simulink model "mylib"  (R2016b)
settings: Solver=FixedStepAuto  StartTime=0.0  StopTime=10.0  RelTol=1e-3  SampleTimeConstraint=STIndependent
settings Model: Creator=Colin  LastModifiedBy=Colin

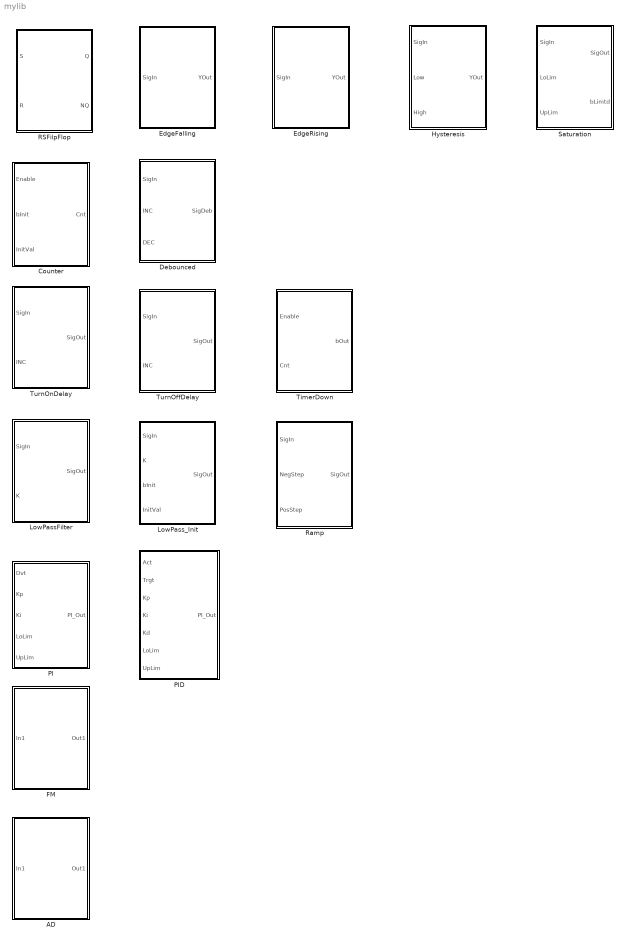
== system mylib ==
  AD : Subsystem
  Counter : Subsystem
  Debounced : Subsystem
  EdgeFalling : Subsystem
  EdgeRising : Subsystem
  FM : Subsystem
  Hysteresis : Subsystem
  LowPassFilter : Subsystem
  LowPass_Init : Subsystem
  PI : Subsystem
  PID : Subsystem
  RSFilpFlop : Subsystem
  Ramp : Subsystem
  Saturation : Subsystem
  TimerDown : Subsystem
  TurnOffDelay : Subsystem
  TurnOnDelay : Subsystem

== system mylib/AD ==
  In1 : Inport
  Out1 : Outport

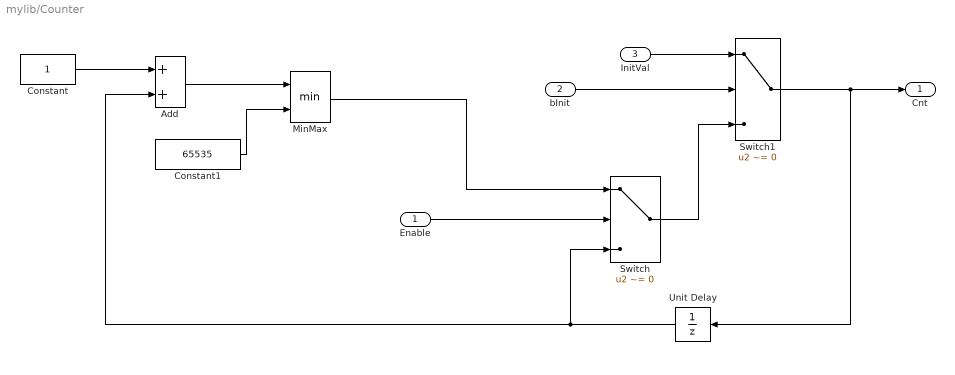
== system mylib/Counter ==
  Enable : Inport
  bInit : Inport  Port=2
  InitVal : Inport  Port=3
  Add : Sum
  Constant : Constant
  Constant1 : Constant  Value=65535
  MinMax : MinMax  Inputs=2
  Switch : Switch  Criteria=u2 ~= 0
  Switch1 : Switch  Criteria=u2 ~= 0
  Unit Delay : UnitDelay  SampleTime=-1
      settings: AttributesFormatString=InitialValue=%<InitialCondition>
  Cnt : Outport
  wires:
  Enable/1 -> Switch/2
  Add/1 -> MinMax/1
  MinMax/1 -> Switch/1
  Constant1/1 -> MinMax/2
  Switch1/1 -> Unit Delay/1, Cnt/1
  bInit/1 -> Switch1/2
  InitVal/1 -> Switch1/1
  Switch/1 -> Switch1/3
  Constant/1 -> Add/1
  Unit Delay/1 -> Switch/3, Add/2

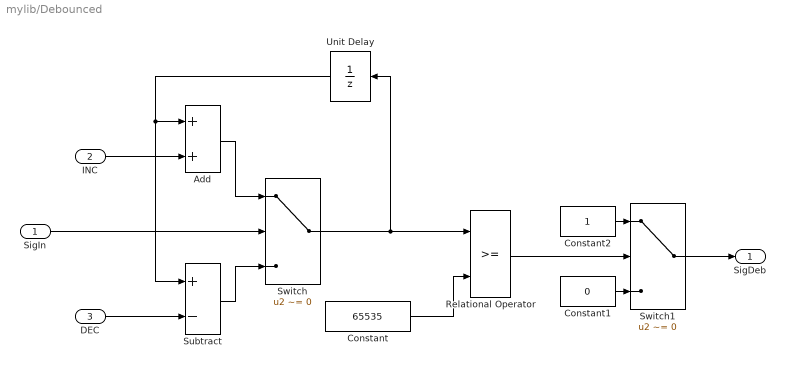
== system mylib/Debounced ==
  SigIn : Inport  OutDataTypeStr=boolean
  INC : Inport  Port=2
  DEC : Inport  Port=3
  Add : Sum
  Constant : Constant  Value=65535
  Constant1 : Constant  Value=0  OutDataTypeStr=boolean
  Constant2 : Constant  OutDataTypeStr=boolean
  Relational Operator : RelationalOperator  OutDataTypeStr=boolean  RndMeth=Simplest
  Subtract : Sum  Inputs=+-
  Switch : Switch  Criteria=u2 ~= 0
  Switch1 : Switch  Criteria=u2 ~= 0
  Unit Delay : UnitDelay  SampleTime=-1
      settings: AttributesFormatString=InitialValue=%<InitialCondition>
  SigDeb : Outport  OutDataTypeStr=boolean
  wires:
  SigIn/1 -> Switch/2
  Switch/1 -> Unit Delay/1, Relational Operator/1
  Constant/1 -> Relational Operator/2
  Relational Operator/1 -> Switch1/2
  Switch1/1 -> SigDeb/1
  Constant1/1 -> Switch1/3
  Constant2/1 -> Switch1/1
  INC/1 -> Add/2
  Unit Delay/1 -> Subtract/1, Add/1
  Add/1 -> Switch/1
  Subtract/1 -> Switch/3
  DEC/1 -> Subtract/2

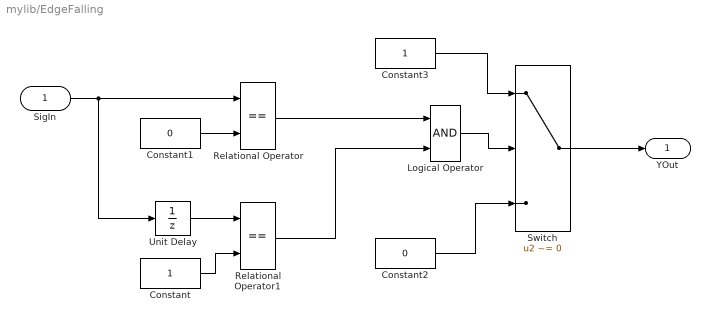
== system mylib/EdgeFalling ==
  SigIn : Inport  OutDataTypeStr=boolean
  Constant : Constant  OutDataTypeStr=boolean
  Constant1 : Constant  Value=0  OutDataTypeStr=boolean
  Constant2 : Constant  Value=0  OutDataTypeStr=boolean
  Constant3 : Constant  OutDataTypeStr=boolean
  Logical Operator : Logic  AllPortsSameDT=off  OutDataTypeStr=boolean
  Relational Operator : RelationalOperator  Operator===  OutDataTypeStr=boolean  RndMeth=Simplest
  Relational Operator1 : RelationalOperator  Operator===  OutDataTypeStr=boolean  RndMeth=Simplest
  Switch : Switch  Criteria=u2 ~= 0
  Unit Delay : UnitDelay  SampleTime=-1
      settings: AttributesFormatString=InitialValue=%<InitialCondition>
  YOut : Outport  OutDataTypeStr=boolean
  wires:
  Logical Operator/1 -> Switch/2
  Switch/1 -> YOut/1
  SigIn/1 -> Unit Delay/1, Relational Operator/1
  Constant1/1 -> Relational Operator/2
  Constant/1 -> Relational Operator1/2
  Unit Delay/1 -> Relational Operator1/1
  Relational Operator/1 -> Logical Operator/1
  Relational Operator1/1 -> Logical Operator/2
  Constant2/1 -> Switch/3
  Constant3/1 -> Switch/1

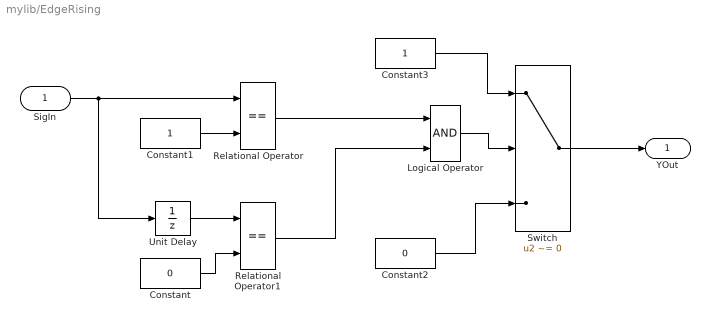
== system mylib/EdgeRising ==
  SigIn : Inport  OutDataTypeStr=boolean
  Constant : Constant  Value=0  OutDataTypeStr=boolean
  Constant1 : Constant  OutDataTypeStr=boolean
  Constant2 : Constant  Value=0  OutDataTypeStr=boolean
  Constant3 : Constant  OutDataTypeStr=boolean
  Logical Operator : Logic  AllPortsSameDT=off  OutDataTypeStr=boolean
  Relational Operator : RelationalOperator  Operator===  OutDataTypeStr=boolean  RndMeth=Simplest
  Relational Operator1 : RelationalOperator  Operator===  OutDataTypeStr=boolean  RndMeth=Simplest
  Switch : Switch  Criteria=u2 ~= 0
  Unit Delay : UnitDelay  SampleTime=-1
      settings: AttributesFormatString=InitialValue=%<InitialCondition>
  YOut : Outport  OutDataTypeStr=boolean
  wires:
  Logical Operator/1 -> Switch/2
  Switch/1 -> YOut/1
  SigIn/1 -> Unit Delay/1, Relational Operator/1
  Constant1/1 -> Relational Operator/2
  Constant/1 -> Relational Operator1/2
  Unit Delay/1 -> Relational Operator1/1
  Relational Operator/1 -> Logical Operator/1
  Relational Operator1/1 -> Logical Operator/2
  Constant2/1 -> Switch/3
  Constant3/1 -> Switch/1

== system mylib/FM ==
  In1 : Inport
  Out1 : Outport

== system mylib/Hysteresis ==
  SigIn : Inport
  Low : Inport  Port=2
  High : Inport  Port=3
  Constant : Constant  OutDataTypeStr=boolean
  Constant1 : Constant  Value=0  OutDataTypeStr=boolean
  Delay : Delay  DelayLength=1  InitialCondition=0
      settings: AttributesFormatString=InitialValue=%<InitialCondition>
  Relational Operator : RelationalOperator  Operator=>  OutDataTypeStr=boolean  RndMeth=Nearest  InputSameDT=on
  Relational Operator1 : RelationalOperator  Operator=<  OutDataTypeStr=boolean  RndMeth=Nearest  InputSameDT=on
  Switch : Switch  Criteria=u2 ~= 0  InputSameDT=on
  Switch1 : Switch  Criteria=u2 ~= 0  InputSameDT=on
  YOut : Outport  OutDataTypeStr=boolean
  wires:
  SigIn/1 -> Relational Operator/1, Relational Operator1/1
  High/1 -> Relational Operator/2
  Relational Operator/1 -> Switch/2
  Constant/1 -> Switch/1
  Switch1/1 -> Switch/3
  Relational Operator1/1 -> Switch1/2
  Low/1 -> Relational Operator1/2
  Constant1/1 -> Switch1/1
  Switch/1 -> YOut/1, Delay/1
  Delay/1 -> Switch1/3

== system mylib/LowPassFilter ==
  SigIn : Inport  SampleTime=0.01
  K : Inport  Port=2  SampleTime=0.01
  Product : Product
  Subtract1 : Sum  Inputs=+-
  Sum : Sum  Inputs=+|+
  Unit Delay : UnitDelay  SampleTime=-1
      settings: AttributesFormatString=InitialValue=%<InitialCondition>
  SigOut : Outport  SampleTime=0.01
  wires:
  K/1 -> Product/1
  SigIn/1 -> Subtract1/1
  Unit Delay/1 -> Sum/2, Subtract1/2
  Subtract1/1 -> Product/2
  Product/1 -> Sum/1
  Sum/1 -> Unit Delay/1, SigOut/1

== system mylib/LowPass_Init ==
  SigIn : Inport  SampleTime=0.01
  K : Inport  Port=2  SampleTime=0.01
  bInit : Inport  Port=3  SampleTime=0.01
  InitVal : Inport  Port=4  SampleTime=0.01
  Product : Product
  Subtract1 : Sum  Inputs=+-
  Sum : Sum  Inputs=+|+
  Switch : Switch  Criteria=u2 ~= 0
  Unit Delay : UnitDelay  SampleTime=-1
      settings: AttributesFormatString=InitialValue=%<InitialCondition>
  SigOut : Outport  SampleTime=0.01
  wires:
  K/1 -> Product/1
  SigIn/1 -> Subtract1/1
  Unit Delay/1 -> Sum/2, Subtract1/2
  Subtract1/1 -> Product/2
  Product/1 -> Sum/1
  Sum/1 -> Switch/3
  Switch/1 -> Unit Delay/1, SigOut/1
  bInit/1 -> Switch/2
  InitVal/1 -> Switch/1

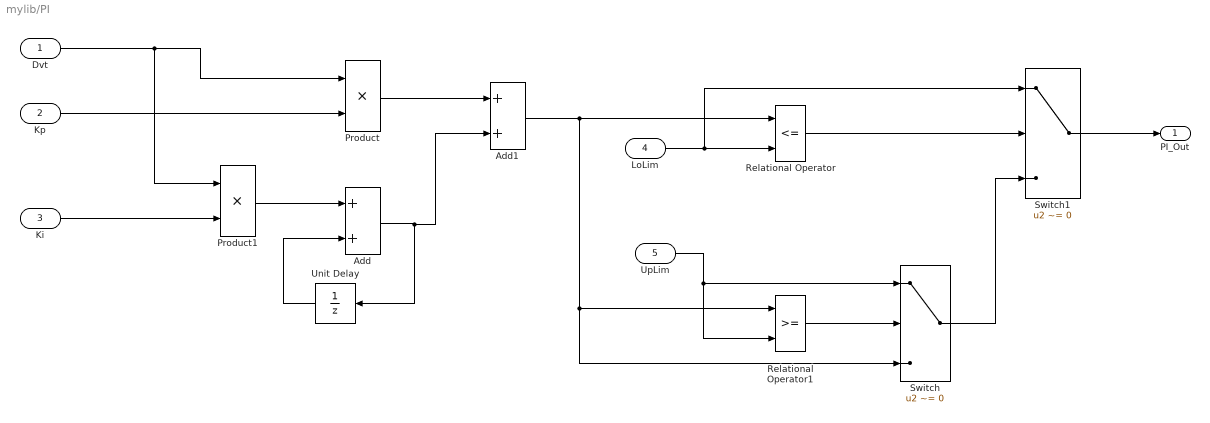
== system mylib/PI ==
  Dvt : Inport
  Kp : Inport  Port=2
  Ki : Inport  Port=3
  LoLim : Inport  Port=4
  UpLim : Inport  Port=5
  Add : Sum
  Add1 : Sum
  Product : Product
  Product1 : Product
  Relational Operator : RelationalOperator  Operator=<=  OutDataTypeStr=boolean  RndMeth=Simplest  InputSameDT=on
  Relational Operator1 : RelationalOperator  OutDataTypeStr=boolean  RndMeth=Simplest  InputSameDT=on
  Switch : Switch  Criteria=u2 ~= 0
  Switch1 : Switch  Criteria=u2 ~= 0
  Unit Delay : UnitDelay  SampleTime=-1
      settings: AttributesFormatString=InitialValue=%<InitialCondition>
  PI_Out : Outport
  wires:
  Dvt/1 -> Product/1, Product1/1
  Kp/1 -> Product/2
  Ki/1 -> Product1/2
  Product1/1 -> Add/1
  Add/1 -> Add1/2, Unit Delay/1
  Unit Delay/1 -> Add/2
  Product/1 -> Add1/1
  Add1/1 -> Relational Operator/1, Switch/3, Relational Operator1/1
  UpLim/1 -> Relational Operator1/2, Switch/1
  LoLim/1 -> Switch1/1, Relational Operator/2
  Relational Operator/1 -> Switch1/2
  Relational Operator1/1 -> Switch/2
  Switch/1 -> Switch1/3
  Switch1/1 -> PI_Out/1

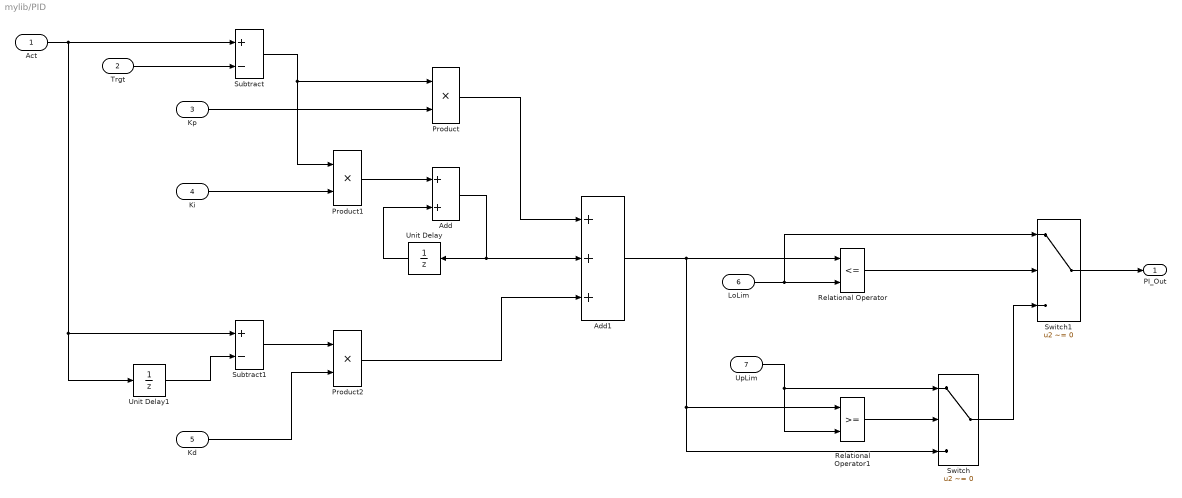
== system mylib/PID ==
  Act : Inport
  Trgt : Inport  Port=2
  Kp : Inport  Port=3
  Ki : Inport  Port=4
  Kd : Inport  Port=5
  LoLim : Inport  Port=6
  UpLim : Inport  Port=7
  Add : Sum
  Add1 : Sum  Inputs=+++
  Product : Product
  Product1 : Product
  Product2 : Product
  Relational Operator : RelationalOperator  Operator=<=  OutDataTypeStr=boolean  RndMeth=Simplest  InputSameDT=on
  Relational Operator1 : RelationalOperator  OutDataTypeStr=boolean  RndMeth=Simplest  InputSameDT=on
  Subtract : Sum  Inputs=+-
  Subtract1 : Sum  Inputs=+-
  Switch : Switch  Criteria=u2 ~= 0
  Switch1 : Switch  Criteria=u2 ~= 0
  Unit Delay : UnitDelay  SampleTime=-1
      settings: AttributesFormatString=InitialValue=%<InitialCondition>
  Unit Delay1 : UnitDelay  SampleTime=-1
      settings: AttributesFormatString=InitialValue=%<InitialCondition>
  PI_Out : Outport
  wires:
  Kp/1 -> Product/2
  Ki/1 -> Product1/2
  Product1/1 -> Add/1
  Add/1 -> Unit Delay/1, Add1/2
  Unit Delay/1 -> Add/2
  Product/1 -> Add1/1
  Add1/1 -> Switch/3, Relational Operator1/1, Relational Operator/1
  UpLim/1 -> Relational Operator1/2, Switch/1
  LoLim/1 -> Switch1/1, Relational Operator/2
  Relational Operator/1 -> Switch1/2
  Relational Operator1/1 -> Switch/2
  Switch/1 -> Switch1/3
  Switch1/1 -> PI_Out/1
  Act/1 -> Unit Delay1/1, Subtract1/1, Subtract/1
  Trgt/1 -> Subtract/2
  Subtract/1 -> Product1/1, Product/1
  Unit Delay1/1 -> Subtract1/2
  Subtract1/1 -> Product2/1
  Kd/1 -> Product2/2
  Product2/1 -> Add1/3

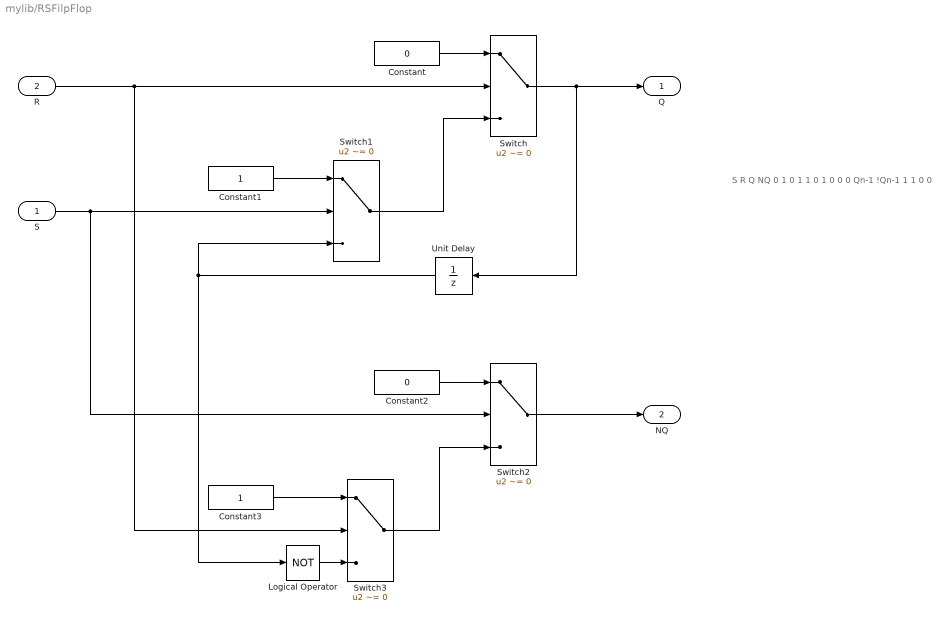
== system mylib/RSFilpFlop ==
  note: S
      | R
      | Q
      | NQ
      |
      | 0
      | 1
      | 0
      | 1
      |
      | 1
      | 0
      | 1
      | 0
      |
      | 0
      | 0
      | Qn-1
      | !Qn-1
      |
      | 1
      | 1
      | 0
      | 0
  S : Inport
  R : Inport  Port=2
  Constant : Constant  Value=0
  Constant1 : Constant
  Constant2 : Constant  Value=0
  Constant3 : Constant
  Logical Operator : Logic  Operator=NOT  AllPortsSameDT=off  OutDataTypeStr=boolean
  Switch{,1..3} (4 alike) : Switch  Criteria=u2 ~= 0
  Unit Delay : UnitDelay  SampleTime=-1
  Q : Outport
  NQ : Outport  Port=2
  wires:
  R/1 -> Switch3/2, Switch/2
  Constant/1 -> Switch/1
  Switch/1 -> Unit Delay/1, Q/1
  S/1 -> Switch2/2, Switch1/2
  Constant1/1 -> Switch1/1
  Switch1/1 -> Switch/3
  Unit Delay/1 -> Switch1/3, Logical Operator/1
  Switch2/1 -> NQ/1
  Constant2/1 -> Switch2/1
  Switch3/1 -> Switch2/3
  Constant3/1 -> Switch3/1
  Logical Operator/1 -> Switch3/3

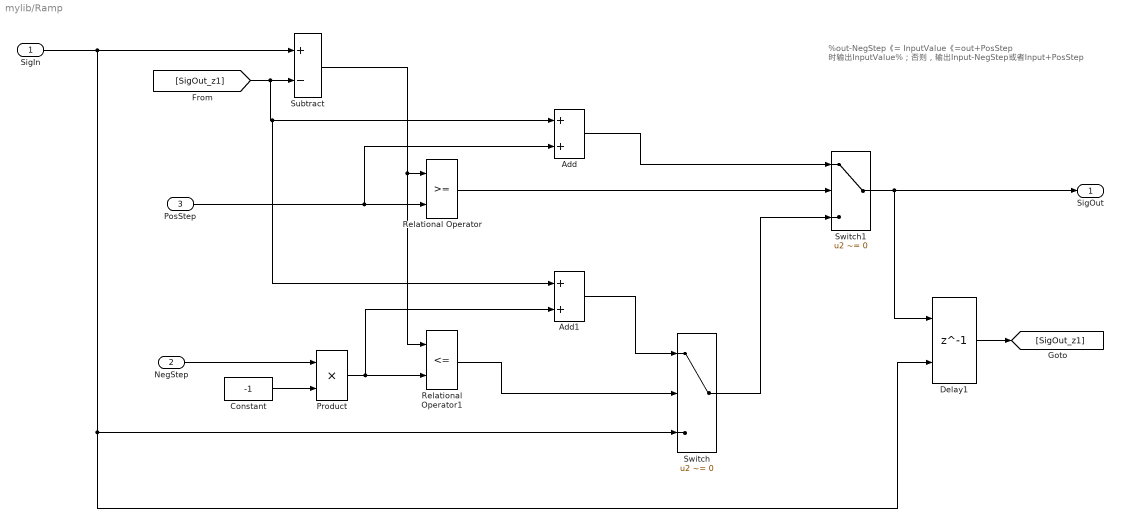
== system mylib/Ramp ==
  note: %out-NegStep《= InputValue《=out+PosStep
      | 时输出InputValue%；否则，输出Input-NegStep或者Input+PosStep
  SigIn : Inport
  NegStep : Inport  Port=2
  PosStep : Inport  Port=3
  Add : Sum
  Add1 : Sum
  Constant : Constant  Value=-1
  Delay1 : Delay  DelayLength=1  InitialConditionSource=Input port
      settings: InputPortMap=u0,p4
  Product : Product
  Relational Operator : RelationalOperator  OutDataTypeStr=boolean  RndMeth=Simplest
  Relational Operator1 : RelationalOperator  Operator=<=  OutDataTypeStr=boolean  RndMeth=Simplest
  Subtract : Sum  Inputs=+-
  Switch : Switch  Criteria=u2 ~= 0
  Switch1 : Switch  Criteria=u2 ~= 0
  SigOut : Outport
  wires:
  SigIn/1 -> Delay1/2, Switch/3, Subtract/1
  Subtract/1 -> Relational Operator1/1, Relational Operator/1
  PosStep/1 -> Add/2, Relational Operator/2
  Relational Operator/1 -> Switch1/2
  Switch1/1 -> Delay1/1, SigOut/1
  Add/1 -> Switch1/1
  Relational Operator1/1 -> Switch/2
  NegStep/1 -> Product/1
  Product/1 -> Add1/2, Relational Operator1/2
  Constant/1 -> Product/2
  Switch/1 -> Switch1/3
  Add1/1 -> Switch/1
  Delay1/1 -> [SigOut_z1]
  [SigOut_z1] -> Add1/1, Add/1, Subtract/2

== system mylib/Saturation ==
  SigIn : Inport
  LoLim : Inport  Port=2
  UpLim : Inport  Port=3
  Logical Operator : Logic  Operator=OR  AllPortsSameDT=off  OutDataTypeStr=boolean
  Relational Operator : RelationalOperator  Operator=<=  OutDataTypeStr=boolean  RndMeth=Simplest  InputSameDT=on
  Relational Operator1 : RelationalOperator  OutDataTypeStr=boolean  RndMeth=Simplest  InputSameDT=on
  Switch : Switch  Criteria=u2 ~= 0
  Switch1 : Switch  Criteria=u2 ~= 0
  SigOut : Outport
  bLimtd : Outport  Port=2  OutDataTypeStr=boolean
  wires:
  SigIn/1 -> Relational Operator/1, Switch/3, Relational Operator1/1
  UpLim/1 -> Relational Operator1/2, Switch/1
  LoLim/1 -> Switch1/1, Relational Operator/2
  Relational Operator/1 -> Logical Operator/1, Switch1/2
  Relational Operator1/1 -> Logical Operator/2, Switch/2
  Logical Operator/1 -> bLimtd/1
  Switch/1 -> Switch1/3
  Switch1/1 -> SigOut/1

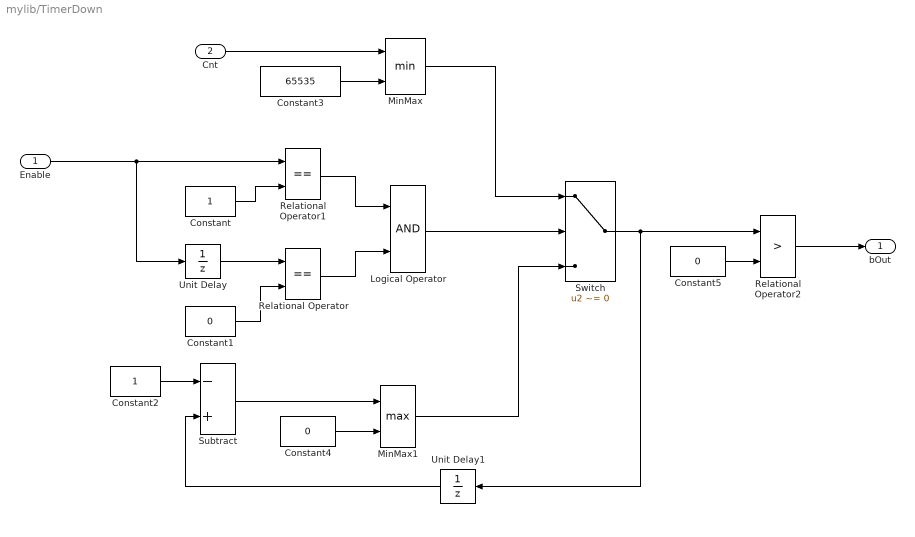
== system mylib/TimerDown ==
  Enable : Inport  OutDataTypeStr=boolean
  Cnt : Inport  Port=2
  Constant : Constant
  Constant1 : Constant  Value=0
  Constant2 : Constant
  Constant3 : Constant  Value=65535
  Constant4 : Constant  Value=0
  Constant5 : Constant  Value=0
  Logical Operator : Logic  AllPortsSameDT=off  OutDataTypeStr=boolean
  MinMax : MinMax  Inputs=2
  MinMax1 : MinMax  Function=max  Inputs=2
  Relational Operator : RelationalOperator  Operator===  OutDataTypeStr=boolean  RndMeth=Simplest
  Relational Operator1 : RelationalOperator  Operator===  OutDataTypeStr=boolean  RndMeth=Simplest
  Relational Operator2 : RelationalOperator  Operator=>  OutDataTypeStr=boolean  RndMeth=Simplest
  Subtract : Sum  Inputs=-+
  Switch : Switch  Criteria=u2 ~= 0
  Unit Delay : UnitDelay  SampleTime=-1
  Unit Delay1 : UnitDelay  SampleTime=-1
      settings: AttributesFormatString=InitialValue=%<InitialCondition>
  bOut : Outport  OutDataTypeStr=boolean
  wires:
  Enable/1 -> Unit Delay/1, Relational Operator1/1
  Unit Delay/1 -> Relational Operator/1
  Constant/1 -> Relational Operator1/2
  Constant1/1 -> Relational Operator/2
  Relational Operator1/1 -> Logical Operator/1
  Relational Operator/1 -> Logical Operator/2
  Logical Operator/1 -> Switch/2
  Cnt/1 -> MinMax/1
  Constant3/1 -> MinMax/2
  MinMax/1 -> Switch/1
  Constant2/1 -> Subtract/1
  Switch/1 -> Relational Operator2/1, Unit Delay1/1
  Unit Delay1/1 -> Subtract/2
  MinMax1/1 -> Switch/3
  Subtract/1 -> MinMax1/1
  Constant4/1 -> MinMax1/2
  Relational Operator2/1 -> bOut/1
  Constant5/1 -> Relational Operator2/2

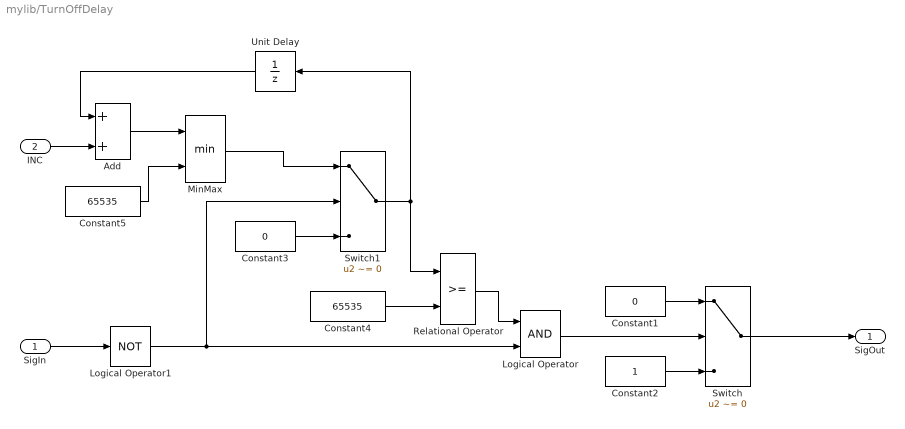
== system mylib/TurnOffDelay ==
  SigIn : Inport  OutDataTypeStr=boolean
  INC : Inport  Port=2
  Add : Sum
  Constant1 : Constant  Value=0
  Constant2 : Constant
  Constant3 : Constant  Value=0
  Constant4 : Constant  Value=65535
  Constant5 : Constant  Value=65535
  Logical Operator : Logic  AllPortsSameDT=off  OutDataTypeStr=boolean
  Logical Operator1 : Logic  Operator=NOT  AllPortsSameDT=off  OutDataTypeStr=boolean
  MinMax : MinMax  Inputs=2
  Relational Operator : RelationalOperator  OutDataTypeStr=boolean  RndMeth=Simplest
  Switch : Switch  Criteria=u2 ~= 0
  Switch1 : Switch  Criteria=u2 ~= 0
  Unit Delay : UnitDelay  SampleTime=-1
      settings: AttributesFormatString=InitialVaule=%<InitialCondition>
  SigOut : Outport  OutDataTypeStr=boolean
  wires:
  Switch/1 -> SigOut/1
  Constant1/1 -> Switch/1
  Constant2/1 -> Switch/3
  SigIn/1 -> Logical Operator1/1
  Logical Operator/1 -> Switch/2
  Constant3/1 -> Switch1/3
  Switch1/1 -> Unit Delay/1, Relational Operator/1
  Constant4/1 -> Relational Operator/2
  Relational Operator/1 -> Logical Operator/1
  Unit Delay/1 -> Add/1
  INC/1 -> Add/2
  Add/1 -> MinMax/1
  Constant5/1 -> MinMax/2
  MinMax/1 -> Switch1/1
  Logical Operator1/1 -> Switch1/2, Logical Operator/2

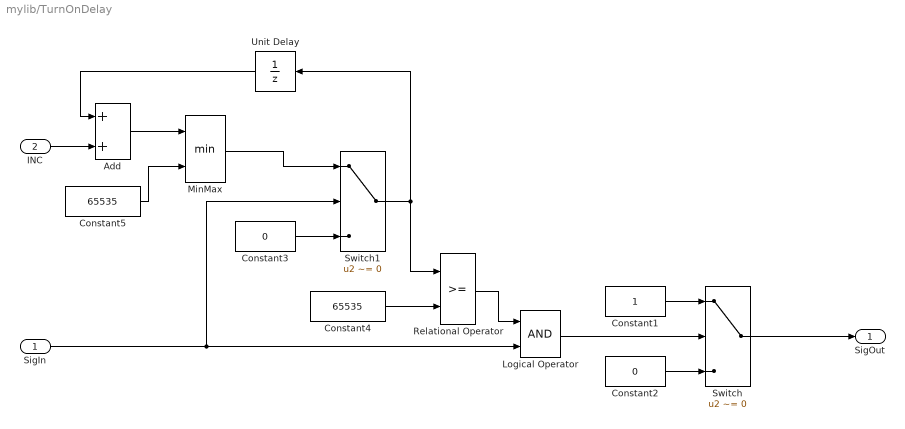
== system mylib/TurnOnDelay ==
  SigIn : Inport  OutDataTypeStr=boolean
  INC : Inport  Port=2
  Add : Sum
  Constant1 : Constant
  Constant2 : Constant  Value=0
  Constant3 : Constant  Value=0
  Constant4 : Constant  Value=65535
  Constant5 : Constant  Value=65535
  Logical Operator : Logic  AllPortsSameDT=off  OutDataTypeStr=boolean
  MinMax : MinMax  Inputs=2
  Relational Operator : RelationalOperator  OutDataTypeStr=boolean  RndMeth=Simplest
  Switch : Switch  Criteria=u2 ~= 0
  Switch1 : Switch  Criteria=u2 ~= 0
  Unit Delay : UnitDelay  SampleTime=-1
      settings: AttributesFormatString=InitialValue=%<InitialCondition>
  SigOut : Outport  OutDataTypeStr=boolean
  wires:
  Switch/1 -> SigOut/1
  Constant1/1 -> Switch/1
  Constant2/1 -> Switch/3
  SigIn/1 -> Switch1/2, Logical Operator/2
  Logical Operator/1 -> Switch/2
  Constant3/1 -> Switch1/3
  Switch1/1 -> Unit Delay/1, Relational Operator/1
  Constant4/1 -> Relational Operator/2
  Relational Operator/1 -> Logical Operator/1
  Unit Delay/1 -> Add/1
  INC/1 -> Add/2
  Add/1 -> MinMax/1
  Constant5/1 -> MinMax/2
  MinMax/1 -> Switch1/1
